simulink model "MyECUModel_OLD"  (R2022a)
settings: Solver=FixedStepAuto  StartTime=0.0  StopTime=1  FixedStep=0.0001  RelTol=1e-3
model workspace (MAT data in the model file):
  rpm = 3000
values from neighbouring files (symbols this model uses):
  AFR = 9.75    [MyECUModel_OLD_Params.m]
  engine_displacement = 0.000599    [MyECUModel_OLD_Params.m]
  fuel_mass_flow_rate = 1    [MyECUModel_OLD_Params.m]
  ignition_1 = 160    [MyECUModel_OLD_Params.m]
  ignition_2 = 250    [MyECUModel_OLD_Params.m]
  ignition_3 = 340    [MyECUModel_OLD_Params.m]
  ignition_4 = 70    [MyECUModel_OLD_Params.m]
  ignition_dwell_time = 0.003    [MyECUModel_OLD_Params.m]
  inj_valve_open_time = 1.134    [MyECUModel_OLD_Params.m]
  injection_duration = 24    [MyECUModel_OLD_Params.m]
  injection_start_1 = 120    [MyECUModel_OLD_Params.m]
  injection_start_2 = 210    [MyECUModel_OLD_Params.m]
  injection_start_3 = 300    [MyECUModel_OLD_Params.m]
  injection_start_4 = 30    [MyECUModel_OLD_Params.m]
  intake_air_temp = 300    [MyECUModel_OLD_Params.m]
  manifold_pressure = 100000    [MyECUModel_OLD_Params.m]
  volumetric_efficiency = 1    [MyECUModel_OLD_Params.m]
libraries: simulink x14
settings Model: Creator=feyzi  LastModifiedBy=feyzi
settings DebuggingCC: UnconnectedInputMsg=warning  UnconnectedOutputMsg=warning  UnconnectedLineMsg=warning
settings HardwareCC: ProdBitPerLong=64  ProdLargestAtomicFloat=None  ProdHWDeviceType=AMD->Athlon 64
settings RTWCC: DLArmComputeVersion=19.05

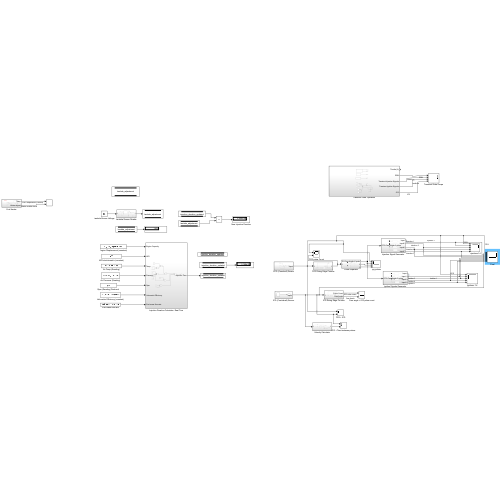
[thumbnail: Simulink's stored preview of the top-level diagram]
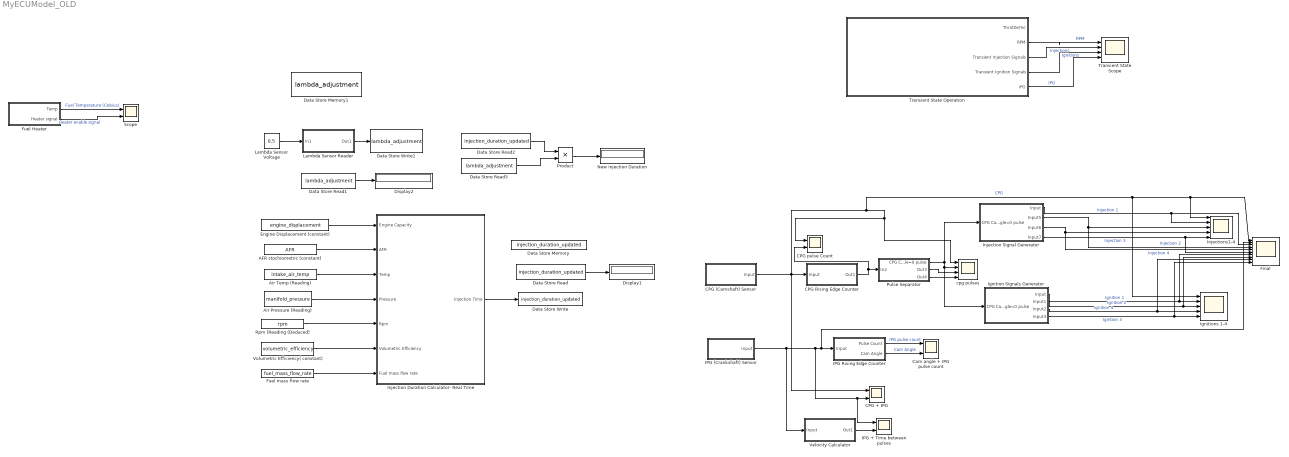
== system MyECUModel_OLD ==
  AFR stochiometric (constant) : Constant  Value=AFR
  Air Pressure (Reading) : Constant  Value=manifold_pressure
  Air Temp (Reading) : Constant  Value=intake_air_temp
  CPG (Camshaft) Sensor : Subsystem
  CPG + IPG : Scope  NumInputPorts=2
  CPG Rising Edge Counter : Subsystem
  CPG pulse Count : Scope  NumInputPorts=2
  Cam angle + IPG pulse count : Scope  NumInputPorts=2
  Data Store Memory : DataStoreMemory  DataStoreName=injection_duration_updated  ReadBeforeWriteMsg=warning  WriteAfterWriteMsg=warning  WriteAfterReadMsg=warning  ShowAdditionalParam=off
  Data Store Memory1 : DataStoreMemory  DataStoreName=lambda_adjustment  ReadBeforeWriteMsg=warning  WriteAfterWriteMsg=warning  WriteAfterReadMsg=warning  ShowAdditionalParam=off
  Data Store Read : DataStoreRead  DataStoreName=injection_duration_updated  IndexOptions=Index vector (dialog)  Indices=1  OutputSizes=1
  Data Store Read1 : DataStoreRead  DataStoreName=lambda_adjustment  IndexOptions=Index vector (dialog)  Indices=1  OutputSizes=1
  Data Store Read2 : DataStoreRead  DataStoreName=injection_duration_updated  IndexOptions=Index vector (dialog)  Indices=1  OutputSizes=1
  Data Store Read3 : DataStoreRead  DataStoreName=lambda_adjustment  IndexOptions=Index vector (dialog)  Indices=1  OutputSizes=1
  Data Store Write : DataStoreWrite  DataStoreName=injection_duration_updated  IndexOptions=Index vector (dialog)  Indices=1  OutputSizes=1
  Data Store Write1 : DataStoreWrite  DataStoreName=lambda_adjustment  IndexOptions=Index vector (dialog)  Indices=1  OutputSizes=1
  Display1 : Display
  Display2 : Display
  Engine Displacement (constant) : Constant  Value=engine_displacement
  Final : Scope  NumInputPorts=10
  Fuel Heater : Subsystem
  Fuel mass flow rate : Constant  Value=fuel_mass_flow_rate
  IPG (Crankshaft) Sensor : Subsystem
  IPG + Time between pulses : Scope  NumInputPorts=2
  IPG Rising Edge Counter : Subsystem
  Ignition Signals Generator : Subsystem
  Ignitions 1-4 : Scope  NumInputPorts=5
  Injection Duration Calculator- Real Time : Subsystem
  Injection Signal Generator : Subsystem
  Injections1-4 : Scope  NumInputPorts=5
  Lambda Sensor Reader : Subsystem
  Lambda Sensor Voltage : Constant  Value=0.5
  New Injection Duration : Display
  Product : Product
  Pulse Separator : Subsystem
  Rpm (Reading (Deduced) : Constant  Value=rpm
  Scope : Scope  NumInputPorts=2
  Transient State Operation : Subsystem
  Transient State Scope : Scope  NumInputPorts=4
  Velocity Calculator : Subsystem
  Volumetric Efficiency( constant) : Constant  Value=volumetric_efficiency
  cpg pulses : Scope  NumInputPorts=4
  wires:
  IPG (Crankshaft) Sensor/1(Input) -> IPG Rising Edge Counter/1(Input), Final/2, CPG + IPG/2, IPG + Time between pulses/1, Velocity Calculator/1(Input)
  CPG (Camshaft) Sensor/1(Input) -> Final/1, Injections1-4/1, Ignitions 1-4/1, cpg pulses/1, CPG pulse Count/1, CPG Rising Edge Counter/1(Input), CPG + IPG/1  "CPG"
  CPG Rising Edge Counter/1(Out1) -> Pulse Separator/1(In2), CPG pulse Count/2
  Pulse Separator/1(CPG Cam Angle=0 pulse) -> Ignition Signals Generator/1(CPG Cam Angle=0 pulse), cpg pulses/2, Injection Signal Generator/1(CPG Cam Angle=0 pulse)
  Pulse Separator/2(Out3) -> cpg pulses/3
  Pulse Separator/3(Out4) -> cpg pulses/4
  Engine Displacement (constant)/1 -> Injection Duration Calculator- Real Time/1(Engine Capacity)
  AFR stochiometric (constant)/1 -> Injection Duration Calculator- Real Time/2(AFR)
  Air Temp (Reading)/1 -> Injection Duration Calculator- Real Time/3(Temp)
  Air Pressure (Reading)/1 -> Injection Duration Calculator- Real Time/4(Pressure)
  Injection Signal Generator/3(Input6) -> Final/5, Injections1-4/4  "Injection 4"
  Injection Signal Generator/2(Input5) -> Injections1-4/3, Final/4  "Injection 2"
  Injection Signal Generator/4(Input7) -> Injections1-4/5, Final/6  "Injection 3"
  Ignition Signals Generator/1(Input) -> Final/7, Ignitions 1-4/2  "Ignition 1"
  Ignition Signals Generator/2(Input1) -> Final/8, Ignitions 1-4/3  "Ignition 2"
  Ignition Signals Generator/3(Input2) -> Final/9, Ignitions 1-4/4  "Ignition 4"
  Ignition Signals Generator/4(Input3) -> Final/10, Ignitions 1-4/5  "Ignition 3"
  Injection Signal Generator/1(Input) -> Injections1-4/2, Final/3  "Injection 1"
  Rpm (Reading (Deduced)/1 -> Injection Duration Calculator- Real Time/5(Rpm)
  Volumetric Efficiency( constant)/1 -> Injection Duration Calculator- Real Time/6(Volumetric Efficiency)
  Fuel mass flow rate/1 -> Injection Duration Calculator- Real Time/7(Fuel mass flow rate)
  Injection Duration Calculator- Real Time/1(Injection Time) -> Data Store Write/1
  IPG Rising Edge Counter/2(Cam Angle) -> Cam angle + IPG pulse count/2  "Cam Angle"
  IPG Rising Edge Counter/1(Pulse Count) -> Cam angle + IPG pulse count/1  "IPG pulse count"
  Data Store Read/1 -> Display1/1
  Lambda Sensor Voltage/1 -> Lambda Sensor Reader/1(In1)
  Lambda Sensor Reader/1(Out1) -> Data Store Write1/1
  Data Store Read1/1 -> Display2/1
  Data Store Read2/1 -> Product/1
  Data Store Read3/1 -> Product/2
  Product/1 -> New Injection Duration/1
  Velocity Calculator/1(Out1) -> IPG + Time between pulses/2
  Transient State Operation/2(RPM) -> Transient State Scope/1  "RPM"
  Transient State Operation/3(Transient Injection Signals) -> Transient State Scope/2  "Injections"
  Transient State Operation/4(Transient Ignition Signals) -> Transient State Scope/3  "Ignitions"
  Transient State Operation/5(ıPG) -> Transient State Scope/4  "IPG"
  Fuel Heater/1(Temp) -> Scope/1  "Fuel Temperature (Celsius)"
  Fuel Heater/2(Heater signal) -> Scope/2  "Heater enable signal"

== system MyECUModel_OLD/CPG (Camshaft) Sensor ==
  Peak 2(Ref) : DiscretePulseGenerator  PulseType=Time based  Period=1  PulseWidth=5  PhaseDelay=0.1
  Peak 3 (TDC- before Power) : DiscretePulseGenerator  PulseType=Time based  Period=1  PulseWidth=5  PhaseDelay=0.5
  Peak1(cycle start - injection TDC) : DiscretePulseGenerator  PulseType=Time based  Period=1  PulseWidth=5
  Sum : Sum  Inputs=|+++  InputSameDT=on
  Unit Delay1 : UnitDelay  SampleTime=-1  HasFrameUpgradeWarning=on
  Input : Outport
  wires:
  Sum/1 -> Unit Delay1/1
  Peak1(cycle start - injection TDC)/1 -> Sum/1
  Peak 2(Ref)/1 -> Sum/2
  Peak 3 (TDC- before Power)/1 -> Sum/3
  Unit Delay1/1 -> Input/1

== system MyECUModel_OLD/CPG Rising Edge Counter ==
  Input : Inport
  Count Resetter : simulink/Logic and Bit Operations/Compare To Constant  relop=>=  const=3.0  OutDataTypeStr=boolean
  Delay : Delay  DelayLength=1
  Detect Rise Positive : simulink/Logic and Bit Operations/Detect Rise Positive  vinit=0  OutDataTypeStr=uint8
  Rising Edge Counter : Subsystem  TreatAsAtomicUnit=on
  Scope : Scope  NumInputPorts=2
  Out1 : Outport
  wires:
  Delay/1 -> Rising Edge Counter/Reset
  Input/1 -> Detect Rise Positive/1, Scope/1  "CPG signal"
  Detect Rise Positive/1 -> Rising Edge Counter/1(In1)  "Rising Edge Detected"
  Count Resetter/1 -> Delay/1
  Rising Edge Counter/1(Out1) -> Out1/1, Scope/2, Count Resetter/1  "CPG Pulse Count"

== system MyECUModel_OLD/Fuel Heater ==
  Ramp : simulink/Sources/Ramp  slope=20  start=0.5  InitialOutput=0
  Ramp1 : simulink/Sources/Ramp  slope=-20  start=2.5  InitialOutput=0
  Step1 : Step  Time=0  Before=30  After=30  SampleTime=0
  Step2 : Step  Time=0.5  SampleTime=0
  Step3 : Step  Time=2.5  After=-1  SampleTime=0
  Sum : Sum  Inputs=|+++
  Sum1 : Sum  Inputs=|++
  Temp : Outport
  Heater signal : Outport  Port=2
  wires:
  ? -> ?
  Step1/1 -> Sum/1
  Ramp/1 -> Sum/2
  Sum/1 -> Temp/1
  Ramp1/1 -> Sum/3
  Step2/1 -> Sum1/2
  Step3/1 -> Sum1/1
  Sum1/1 -> Heater signal/1

== system MyECUModel_OLD/IPG (Crankshaft) Sensor ==
  Pulse Generator : DiscretePulseGenerator  PulseType=Time based  Period=0.042  PulseWidth=5
  Input : Outport
  wires:
  Pulse Generator/1 -> Input/1

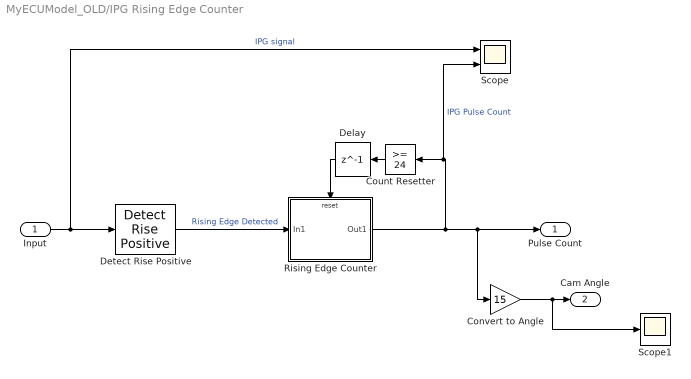
== system MyECUModel_OLD/IPG Rising Edge Counter ==
  Input : Inport
  Convert to Angle : Gain  Gain=15
  Count Resetter : simulink/Logic and Bit Operations/Compare To Constant  relop=>=  const=24  OutDataTypeStr=boolean
  Delay : Delay  DelayLength=1
  Detect Rise Positive : simulink/Logic and Bit Operations/Detect Rise Positive  vinit=0  OutDataTypeStr=uint8
  Rising Edge Counter : Subsystem  TreatAsAtomicUnit=on
  Scope : Scope  NumInputPorts=2
  Scope1 : Scope
  Pulse Count : Outport
  Cam Angle : Outport  Port=2
  wires:
  Delay/1 -> Rising Edge Counter/Reset
  Input/1 -> Detect Rise Positive/1, Scope/1  "IPG signal"
  Detect Rise Positive/1 -> Rising Edge Counter/1(In1)  "Rising Edge Detected"
  Count Resetter/1 -> Delay/1
  Rising Edge Counter/1(Out1) -> Convert to Angle/1, Pulse Count/1, Scope/2, Count Resetter/1  "IPG Pulse Count"
  Convert to Angle/1 -> Scope1/1, Cam Angle/1

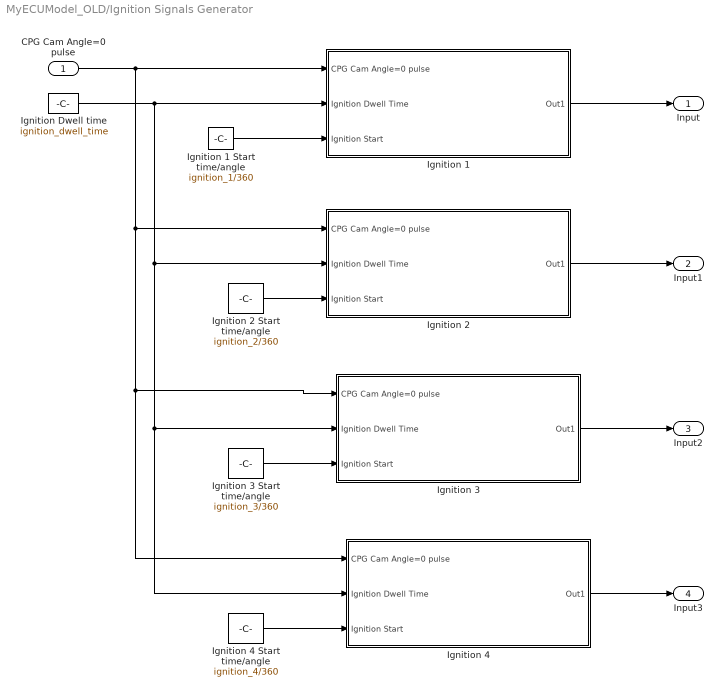
== system MyECUModel_OLD/Ignition Signals Generator ==
  CPG Cam Angle=0 pulse : Inport
  Ignition 1 : Subsystem
  Ignition 1 Start time/angle : Constant  Value=ignition_1/360
  Ignition 2 : Subsystem
  Ignition 2 Start time/angle : Constant  Value=ignition_2/360
  Ignition 3 : Subsystem
  Ignition 3 Start time/angle : Constant  Value=ignition_3/360
  Ignition 4 : Subsystem
  Ignition 4 Start time/angle : Constant  Value=ignition_4/360
  Ignition Dwell time : Constant  Value=ignition_dwell_time
  Input : Outport
  Input1 : Outport  Port=2
  Input2 : Outport  Port=3
  Input3 : Outport  Port=4
  wires:
  CPG Cam Angle=0 pulse/1 -> Ignition 2/1(CPG Cam Angle=0 pulse), Ignition 4/1(CPG Cam Angle=0 pulse), Ignition 3/1(CPG Cam Angle=0 pulse), Ignition 1/1(CPG Cam Angle=0 pulse)
  Ignition Dwell time/1 -> Ignition 2/2(Ignition Dwell Time), Ignition 4/2(Ignition Dwell Time), Ignition 3/2(Ignition Dwell Time), Ignition 1/2(Ignition Dwell Time)
  Ignition 1 Start time/angle/1 -> Ignition 1/3(Ignition Start)
  Ignition 1/1(Out1) -> Input/1
  Ignition 2/1(Out1) -> Input1/1
  Ignition 3/1(Out1) -> Input2/1
  Ignition 4/1(Out1) -> Input3/1
  Ignition 2 Start time/angle/1 -> Ignition 2/3(Ignition Start)
  Ignition 3 Start time/angle/1 -> Ignition 3/3(Ignition Start)
  Ignition 4 Start time/angle/1 -> Ignition 4/3(Ignition Start)

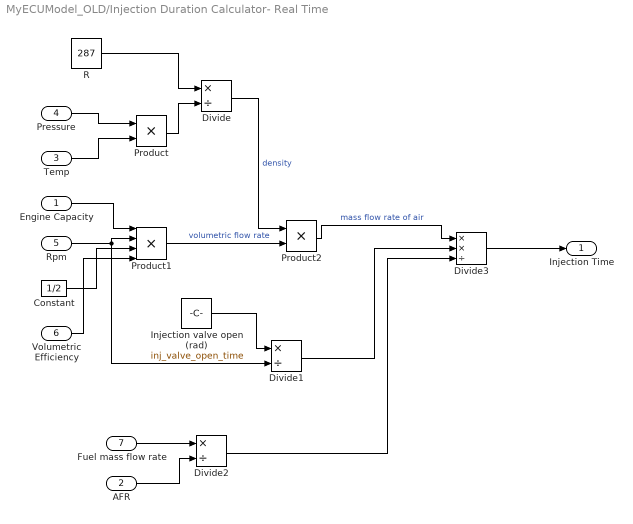
== system MyECUModel_OLD/Injection Duration Calculator- Real Time ==
  Engine Capacity : Inport
  AFR : Inport  Port=2
  Temp : Inport  Port=3
  Pressure : Inport  Port=4
  Rpm : Inport  Port=5
  Volumetric Efficiency : Inport  Port=6
  Fuel mass flow rate : Inport  Port=7
  Constant : Constant  Value=1/2
  Divide : Product  Inputs=*/
  Divide1 : Product  Inputs=*/
  Divide2 : Product  Inputs=*/
  Divide3 : Product  Inputs=**/
  Injection valve open (rad) : Constant  Value=inj_valve_open_time
  Product : Product
  Product1 : Product  Inputs=4
  Product2 : Product
  R : Constant  Value=287
  Injection Time : Outport
  wires:
  Pressure/1 -> Product/1
  Temp/1 -> Product/2
  R/1 -> Divide/1
  Product/1 -> Divide/2
  Divide/1 -> Product2/1  "density"
  Engine Capacity/1 -> Product1/1
  Rpm/1 -> Divide1/2, Product1/2
  Constant/1 -> Product1/3
  Product1/1 -> Product2/2  "volumetric flow rate"
  Product2/1 -> Divide3/1  "mass flow rate of air"
  Injection valve open (rad)/1 -> Divide1/1
  Fuel mass flow rate/1 -> Divide2/1
  AFR/1 -> Divide2/2
  Volumetric Efficiency/1 -> Product1/4
  Divide2/1 -> Divide3/3
  Divide1/1 -> Divide3/2
  Divide3/1 -> Injection Time/1

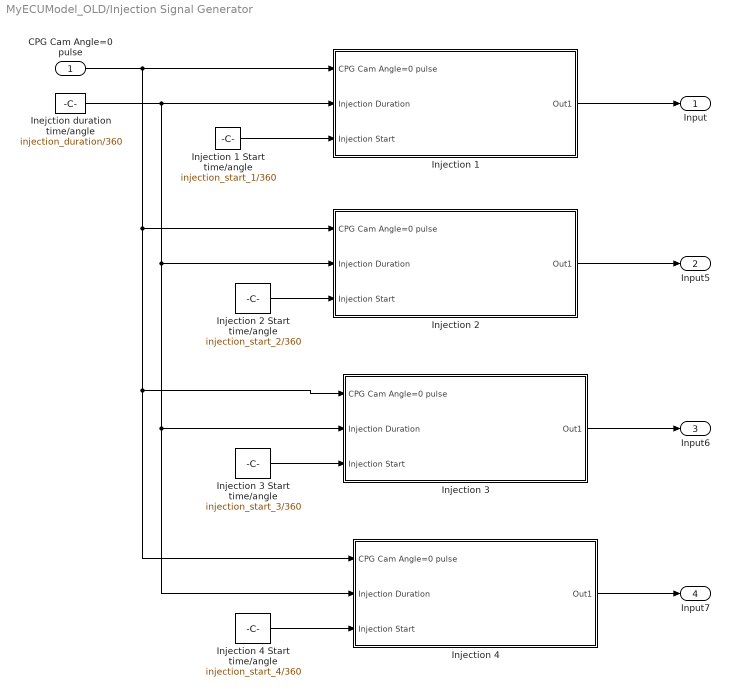
== system MyECUModel_OLD/Injection Signal Generator ==
  CPG Cam Angle=0 pulse : Inport
  Inejction duration time/angle : Constant  Value=injection_duration/360
  Injection 1 : Subsystem
  Injection 1 Start time/angle : Constant  Value=injection_start_1/360
  Injection 2 : Subsystem
  Injection 2 Start time/angle : Constant  Value=injection_start_2/360
  Injection 3 : Subsystem
  Injection 3 Start time/angle : Constant  Value=injection_start_3/360
  Injection 4 : Subsystem
  Injection 4 Start time/angle : Constant  Value=injection_start_4/360
  Input : Outport
  Input5 : Outport  Port=2
  Input6 : Outport  Port=3
  Input7 : Outport  Port=4
  wires:
  CPG Cam Angle=0 pulse/1 -> Injection 3/1(CPG Cam Angle=0 pulse), Injection 4/1(CPG Cam Angle=0 pulse), Injection 2/1(CPG Cam Angle=0 pulse), Injection 1/1(CPG Cam Angle=0 pulse)
  Inejction duration time/angle/1 -> Injection 4/2(Injection Duration), Injection 3/2(Injection Duration), Injection 2/2(Injection Duration), Injection 1/2(Injection Duration)
  Injection 1 Start time/angle/1 -> Injection 1/3(Injection Start)
  Injection 1/1(Out1) -> Input/1
  Injection 2/1(Out1) -> Input5/1
  Injection 3/1(Out1) -> Input6/1
  Injection 4/1(Out1) -> Input7/1
  Injection 2 Start time/angle/1 -> Injection 2/3(Injection Start)
  Injection 3 Start time/angle/1 -> Injection 3/3(Injection Start)
  Injection 4 Start time/angle/1 -> Injection 4/3(Injection Start)

== system MyECUModel_OLD/Lambda Sensor Reader ==
  In1 : Inport
  AFR-Actual : Display
  AFRs : Constant  Value=[19:-0.5:9]
  Constant : Constant  Value=AFR
  Divide : Product  Inputs=/*
  Lookup Table Dynamic : simulink/Lookup Tables/Lookup Table Dynamic  LookUpMeth=Interpolation-Use End Values  OutDataType=fixdt('double')  OutScaling=[]  OutputDataTypeScalingMode=Specify via dialog  OutDataTypeStr=double  DoSatur=off
  Voltages : Constant  Value=[0:0.05:1]
  Out1 : Outport
  wires:
  In1/1 -> Lookup Table Dynamic/1
  Voltages/1 -> Lookup Table Dynamic/2
  AFRs/1 -> Lookup Table Dynamic/3
  Lookup Table Dynamic/1 -> AFR-Actual/1, Divide/2
  Divide/1 -> Out1/1
  Constant/1 -> Divide/1

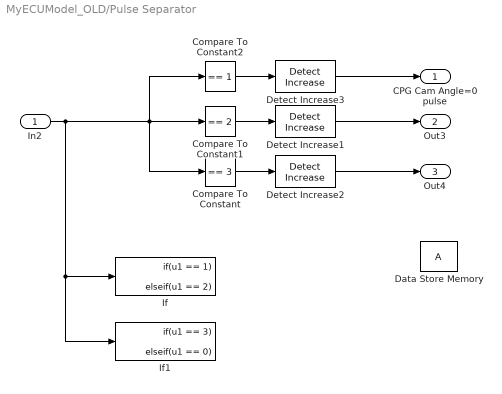
== system MyECUModel_OLD/Pulse Separator ==
  In2 : Inport
  Compare To Constant : simulink/Logic and Bit Operations/Compare To Constant  relop===  const=3  OutDataTypeStr=uint8
  Compare To Constant1 : simulink/Logic and Bit Operations/Compare To Constant  relop===  const=2  OutDataTypeStr=uint8
  Compare To Constant2 : simulink/Logic and Bit Operations/Compare To Constant  relop===  const=1  OutDataTypeStr=uint8
  Data Store Memory : DataStoreMemory  ReadBeforeWriteMsg=warning  WriteAfterWriteMsg=warning  WriteAfterReadMsg=warning  ShareAcrossModelInstances=on  ShowAdditionalParam=off  OutMin=0  OutMax=12
  Detect Increase1 : simulink/Logic and Bit Operations/Detect Increase  vinit=0.0  OutDataTypeStr=uint8
  Detect Increase2 : simulink/Logic and Bit Operations/Detect Increase  vinit=0.0  OutDataTypeStr=uint8
  Detect Increase3 : simulink/Logic and Bit Operations/Detect Increase  vinit=0.0  OutDataTypeStr=uint8
  If : If  IfExpression=u1 == 1  ElseIfExpressions=u1 == 2  ShowElse=off
  If1 : If  IfExpression=u1 == 3  ElseIfExpressions=u1 == 0  ShowElse=off
  CPG Cam Angle=0 pulse : Outport  OutDataTypeStr=uint8
  Out3 : Outport  Port=2
  Out4 : Outport  Port=3
  wires:
  Detect Increase2/1 -> Out4/1
  In2/1 -> If1/1, If/1, Compare To Constant2/1, Compare To Constant/1, Compare To Constant1/1
  Compare To Constant1/1 -> Detect Increase1/1
  Detect Increase1/1 -> Out3/1
  Compare To Constant/1 -> Detect Increase2/1
  Compare To Constant2/1 -> Detect Increase3/1
  Detect Increase3/1 -> CPG Cam Angle=0 pulse/1

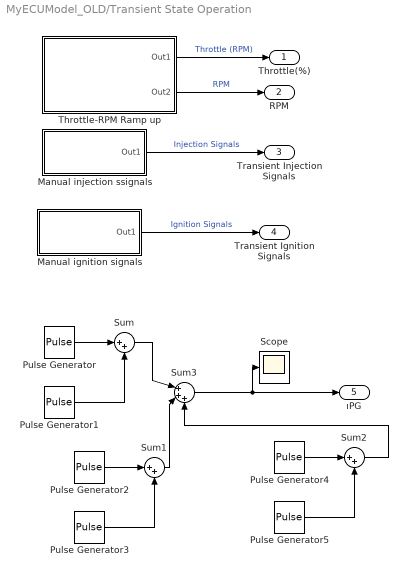
== system MyECUModel_OLD/Transient State Operation ==
  Manual ignition signals : Subsystem
  Manual injection ssignals : Subsystem
  Pulse Generator : DiscretePulseGenerator  PulseType=Time based  Period=0.1  PulseWidth=5
  Pulse Generator1 : DiscretePulseGenerator  PulseType=Time based  Amplitude=-1  Period=0.1  PulseWidth=5  PhaseDelay=1
  Pulse Generator2 : DiscretePulseGenerator  PulseType=Time based  Period=0.08  PulseWidth=5  PhaseDelay=1
  Pulse Generator3 : DiscretePulseGenerator  PulseType=Time based  Amplitude=-1  Period=0.08  PulseWidth=5  PhaseDelay=1.96
  Pulse Generator4 : DiscretePulseGenerator  PulseType=Time based  Period=0.06  PulseWidth=5  PhaseDelay=1.96
  Pulse Generator5 : DiscretePulseGenerator  PulseType=Time based  Amplitude=-1  Period=0.06  PulseWidth=5  PhaseDelay=3
  Scope : Scope
  Sum : Sum  Inputs=|++
  Sum1 : Sum  Inputs=|++
  Sum2 : Sum  Inputs=|++
  Sum3 : Sum  Inputs=|+++
  Throttle-RPM Ramp up : Subsystem
  Throttle(%) : Outport
  RPM : Outport  Port=2
  Transient Injection Signals : Outport  Port=3
  Transient Ignition Signals : Outport  Port=4
  ıPG : Outport  Port=5
  wires:
  Throttle-RPM Ramp up/2(Out2) -> RPM/1  "RPM"
  Throttle-RPM Ramp up/1(Out1) -> Throttle(%)/1  "Throttle (RPM)"
  Manual injection ssignals/1(Out1) -> Transient Injection Signals/1  "Injection Signals"
  Manual ignition signals/1(Out1) -> Transient Ignition Signals/1  "Ignition Signals"
  Pulse Generator/1 -> Sum/1
  Pulse Generator1/1 -> Sum/2
  Sum/1 -> Sum3/1
  Pulse Generator2/1 -> Sum1/1
  Pulse Generator3/1 -> Sum1/2
  Pulse Generator4/1 -> Sum2/1
  Pulse Generator5/1 -> Sum2/2
  Sum2/1 -> Sum3/3
  Sum1/1 -> Sum3/2
  Sum3/1 -> Scope/1, ıPG/1

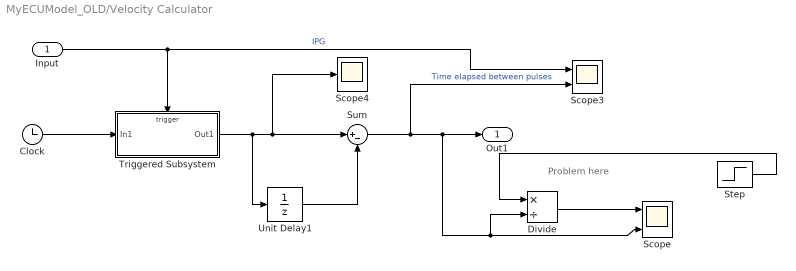
== system MyECUModel_OLD/Velocity Calculator ==
  note: Problem here
  Input : Inport
  Clock : Clock
      settings: Decimation=100
  Divide : Product  Inputs=*/
  Scope : Scope  NumInputPorts=2
  Scope3 : Scope  NumInputPorts=2
  Scope4 : Scope
  Step : Step  Time=0  After=30/12  SampleTime=0
  Sum : Sum  Inputs=|+-
  Triggered Subsystem : Subsystem  TreatAsAtomicUnit=on
  Unit Delay1 : UnitDelay  SampleTime=-1
  Out1 : Outport
  wires:
  Sum/1 -> Scope3/2, Divide/2, Scope/2, Out1/1  "Time elapsed between pulses"
  Input/1 -> Scope3/1, Triggered Subsystem/Trigger  "IPG"
  Unit Delay1/1 -> Sum/2
  Clock/1 -> Triggered Subsystem/1(In1)
  Triggered Subsystem/1(Out1) -> Sum/1, Scope4/1, Unit Delay1/1
  Step/1 -> Divide/1
  Divide/1 -> Scope/1

== system MyECUModel_OLD/CPG Rising Edge Counter/Rising Edge Counter ==
  In1 : Inport
  Reset : ResetPort  DisableCoverage=on
  Memory : Memory
  Sum1 : Sum  Inputs=|++
  Out1 : Outport
  wires:
  Memory/1 -> Sum1/2
  Sum1/1 -> Out1/1, Memory/1
  In1/1 -> Sum1/1

== system MyECUModel_OLD/IPG Rising Edge Counter/Rising Edge Counter ==
  In1 : Inport
  Reset : ResetPort  DisableCoverage=on
  Memory : Memory
  Sum1 : Sum  Inputs=|++
  Out1 : Outport
  wires:
  Memory/1 -> Sum1/2
  Sum1/1 -> Out1/1, Memory/1
  In1/1 -> Sum1/1

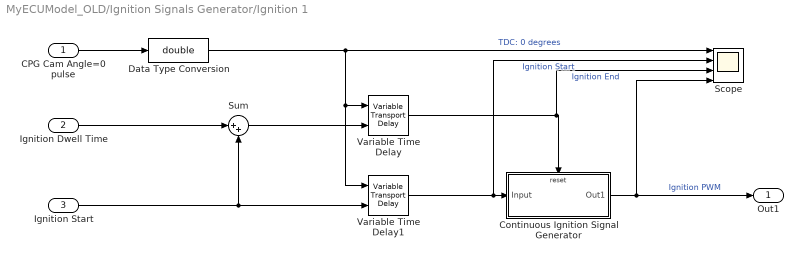
== system MyECUModel_OLD/Ignition Signals Generator/Ignition 1 ==
  CPG Cam Angle=0 pulse : Inport
  Ignition Dwell Time : Inport  Port=2
  Ignition Start : Inport  Port=3
  Continuous Ignition Signal Generator : Subsystem  TreatAsAtomicUnit=on
  Data Type Conversion : DataTypeConversion  OutDataTypeStr=double  SaturateOnIntegerOverflow=off  RndMeth=Floor
  Scope : Scope  NumInputPorts=4
  Sum : Sum  Inputs=|++
  Variable Time Delay : VariableTransportDelay  MaximumDelay=10  MaximumPoints=20480  ZeroDelay=on
  Variable Time Delay1 : VariableTransportDelay  MaximumDelay=10  MaximumPoints=20480  ZeroDelay=on
  Out1 : Outport
  wires:
  Continuous Ignition Signal Generator/1(Out1) -> Scope/4, Out1/1  "Ignition PWM"
  Variable Time Delay/1 -> Scope/3, Continuous Ignition Signal Generator/Reset  "Ignition End"
  Ignition Start/1 -> Sum/2, Variable Time Delay1/2
  CPG Cam Angle=0 pulse/1 -> Data Type Conversion/1
  Variable Time Delay1/1 -> Scope/2, Continuous Ignition Signal Generator/1(Input)  "Ignition Start"
  Data Type Conversion/1 -> Scope/1, Variable Time Delay1/1, Variable Time Delay/1  "TDC: 0 degrees"
  Ignition Dwell Time/1 -> Sum/1
  Sum/1 -> Variable Time Delay/2

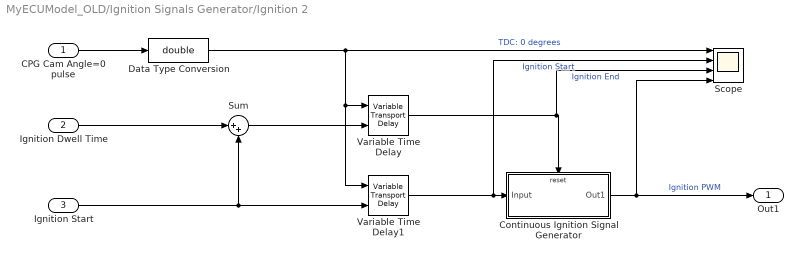
== system MyECUModel_OLD/Ignition Signals Generator/Ignition 2 ==
  CPG Cam Angle=0 pulse : Inport
  Ignition Dwell Time : Inport  Port=2
  Ignition Start : Inport  Port=3
  Continuous Ignition Signal Generator : Subsystem  TreatAsAtomicUnit=on
  Data Type Conversion : DataTypeConversion  OutDataTypeStr=double  SaturateOnIntegerOverflow=off  RndMeth=Floor
  Scope : Scope  NumInputPorts=4
  Sum : Sum  Inputs=|++
  Variable Time Delay : VariableTransportDelay  MaximumDelay=10  MaximumPoints=20480  ZeroDelay=on
  Variable Time Delay1 : VariableTransportDelay  MaximumDelay=10  MaximumPoints=20480  ZeroDelay=on
  Out1 : Outport
  wires:
  Continuous Ignition Signal Generator/1(Out1) -> Scope/4, Out1/1  "Ignition PWM"
  Variable Time Delay/1 -> Scope/3, Continuous Ignition Signal Generator/Reset  "Ignition End"
  Ignition Start/1 -> Sum/2, Variable Time Delay1/2
  CPG Cam Angle=0 pulse/1 -> Data Type Conversion/1
  Variable Time Delay1/1 -> Scope/2, Continuous Ignition Signal Generator/1(Input)  "Ignition Start"
  Data Type Conversion/1 -> Scope/1, Variable Time Delay1/1, Variable Time Delay/1  "TDC: 0 degrees"
  Ignition Dwell Time/1 -> Sum/1
  Sum/1 -> Variable Time Delay/2

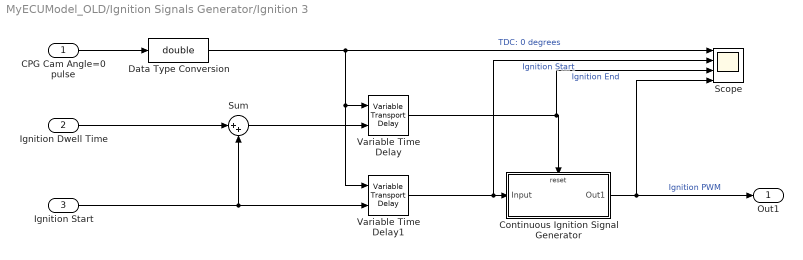
== system MyECUModel_OLD/Ignition Signals Generator/Ignition 3 ==
  CPG Cam Angle=0 pulse : Inport
  Ignition Dwell Time : Inport  Port=2
  Ignition Start : Inport  Port=3
  Continuous Ignition Signal Generator : Subsystem  TreatAsAtomicUnit=on
  Data Type Conversion : DataTypeConversion  OutDataTypeStr=double  SaturateOnIntegerOverflow=off  RndMeth=Floor
  Scope : Scope  NumInputPorts=4
  Sum : Sum  Inputs=|++
  Variable Time Delay : VariableTransportDelay  MaximumDelay=10  MaximumPoints=20480  ZeroDelay=on
  Variable Time Delay1 : VariableTransportDelay  MaximumDelay=10  MaximumPoints=20480  ZeroDelay=on
  Out1 : Outport
  wires:
  Continuous Ignition Signal Generator/1(Out1) -> Scope/4, Out1/1  "Ignition PWM"
  Variable Time Delay/1 -> Scope/3, Continuous Ignition Signal Generator/Reset  "Ignition End"
  Ignition Start/1 -> Sum/2, Variable Time Delay1/2
  CPG Cam Angle=0 pulse/1 -> Data Type Conversion/1
  Variable Time Delay1/1 -> Scope/2, Continuous Ignition Signal Generator/1(Input)  "Ignition Start"
  Data Type Conversion/1 -> Scope/1, Variable Time Delay1/1, Variable Time Delay/1  "TDC: 0 degrees"
  Ignition Dwell Time/1 -> Sum/1
  Sum/1 -> Variable Time Delay/2

== system MyECUModel_OLD/Ignition Signals Generator/Ignition 4 ==
  CPG Cam Angle=0 pulse : Inport
  Ignition Dwell Time : Inport  Port=2
  Ignition Start : Inport  Port=3
  Continuous Ignition Signal Generator : Subsystem  TreatAsAtomicUnit=on
  Data Type Conversion : DataTypeConversion  OutDataTypeStr=double  SaturateOnIntegerOverflow=off  RndMeth=Floor
  Scope : Scope  NumInputPorts=4
  Sum : Sum  Inputs=|++
  Variable Time Delay : VariableTransportDelay  MaximumDelay=10  MaximumPoints=20480  ZeroDelay=on
  Variable Time Delay1 : VariableTransportDelay  MaximumDelay=10  MaximumPoints=20480  ZeroDelay=on
  Out1 : Outport
  wires:
  Continuous Ignition Signal Generator/1(Out1) -> Scope/4, Out1/1  "Ignition PWM"
  Variable Time Delay/1 -> Scope/3, Continuous Ignition Signal Generator/Reset  "Ignition End"
  Ignition Start/1 -> Variable Time Delay1/2, Sum/2
  CPG Cam Angle=0 pulse/1 -> Data Type Conversion/1
  Variable Time Delay1/1 -> Scope/2, Continuous Ignition Signal Generator/1(Input)  "Ignition Start"
  Data Type Conversion/1 -> Scope/1, Variable Time Delay1/1, Variable Time Delay/1  "TDC: 0 degrees"
  Ignition Dwell Time/1 -> Sum/1
  Sum/1 -> Variable Time Delay/2

== system MyECUModel_OLD/Injection Signal Generator/Injection 1 ==
  CPG Cam Angle=0 pulse : Inport
  Injection Duration : Inport  Port=2
  Injection Start : Inport  Port=3
  Continuous Injection Signal Generator : Subsystem  TreatAsAtomicUnit=on
  Data Type Conversion : DataTypeConversion  OutDataTypeStr=double  SaturateOnIntegerOverflow=off  RndMeth=Floor
  Scope : Scope  NumInputPorts=4
  Sum : Sum  Inputs=|++
  Variable Time Delay : VariableTransportDelay  MaximumDelay=10  MaximumPoints=20480  ZeroDelay=on
  Variable Time Delay1 : VariableTransportDelay  MaximumDelay=10  MaximumPoints=30720  ZeroDelay=on
  Out1 : Outport
  wires:
  Continuous Injection Signal Generator/1(Out1) -> Scope/4, Out1/1  "Injection 1 pwm"
  Variable Time Delay/1 -> Scope/3, Continuous Injection Signal Generator/Reset  "Injection 1 end"
  Injection Start/1 -> Sum/2, Variable Time Delay1/2
  CPG Cam Angle=0 pulse/1 -> Data Type Conversion/1
  Variable Time Delay1/1 -> Scope/2, Continuous Injection Signal Generator/1(Input)  "Injection 1 start"
  Data Type Conversion/1 -> Scope/1, Variable Time Delay1/1, Variable Time Delay/1  "TDC: 0 degrees"
  Injection Duration/1 -> Sum/1
  Sum/1 -> Variable Time Delay/2

== system MyECUModel_OLD/Injection Signal Generator/Injection 2 ==
  CPG Cam Angle=0 pulse : Inport
  Injection Duration : Inport  Port=2
  Injection Start : Inport  Port=3
  Continuous Injection Signal Generator : Subsystem  TreatAsAtomicUnit=on
  Data Type Conversion : DataTypeConversion  OutDataTypeStr=double  SaturateOnIntegerOverflow=off  RndMeth=Floor
  Scope : Scope  NumInputPorts=4
  Sum : Sum  Inputs=|++
  Variable Time Delay : VariableTransportDelay  MaximumDelay=10  MaximumPoints=20480  ZeroDelay=on
  Variable Time Delay1 : VariableTransportDelay  MaximumDelay=10  MaximumPoints=30720  ZeroDelay=on
  Out1 : Outport
  wires:
  Continuous Injection Signal Generator/1(Out1) -> Scope/4, Out1/1  "Injection 2 pwm"
  Variable Time Delay/1 -> Scope/3, Continuous Injection Signal Generator/Reset  "Injection 2 end"
  Injection Start/1 -> Sum/2, Variable Time Delay1/2
  CPG Cam Angle=0 pulse/1 -> Data Type Conversion/1
  Variable Time Delay1/1 -> Scope/2, Continuous Injection Signal Generator/1(Input)  "Injection 2 start"
  Data Type Conversion/1 -> Scope/1, Variable Time Delay1/1, Variable Time Delay/1  "TDC: 0 degrees"
  Injection Duration/1 -> Sum/1
  Sum/1 -> Variable Time Delay/2

== system MyECUModel_OLD/Injection Signal Generator/Injection 3 ==
  CPG Cam Angle=0 pulse : Inport
  Injection Duration : Inport  Port=2
  Injection Start : Inport  Port=3
  Continuous Injection Signal Generator : Subsystem  TreatAsAtomicUnit=on
  Data Type Conversion : DataTypeConversion  OutDataTypeStr=double  SaturateOnIntegerOverflow=off  RndMeth=Floor
  Scope : Scope  NumInputPorts=4
  Sum : Sum  Inputs=|++
  Variable Time Delay : VariableTransportDelay  MaximumDelay=10  MaximumPoints=20480  ZeroDelay=on
  Variable Time Delay1 : VariableTransportDelay  MaximumDelay=10  MaximumPoints=20480  ZeroDelay=on
  Out1 : Outport
  wires:
  Continuous Injection Signal Generator/1(Out1) -> Scope/4, Out1/1  "Injection 3 pwm"
  Variable Time Delay/1 -> Scope/3, Continuous Injection Signal Generator/Reset  "Injection 3 end"
  Injection Start/1 -> Sum/2, Variable Time Delay1/2
  CPG Cam Angle=0 pulse/1 -> Data Type Conversion/1
  Variable Time Delay1/1 -> Scope/2, Continuous Injection Signal Generator/1(Input)  "Injection 3 start"
  Data Type Conversion/1 -> Scope/1, Variable Time Delay1/1, Variable Time Delay/1  "TDC: 0 degrees"
  Injection Duration/1 -> Sum/1
  Sum/1 -> Variable Time Delay/2

== system MyECUModel_OLD/Injection Signal Generator/Injection 4 ==
  CPG Cam Angle=0 pulse : Inport
  Injection Duration : Inport  Port=2
  Injection Start : Inport  Port=3
  Continuous Injection Signal Generator : Subsystem  TreatAsAtomicUnit=on
  Data Type Conversion : DataTypeConversion  OutDataTypeStr=double  SaturateOnIntegerOverflow=off  RndMeth=Floor
  Scope : Scope  NumInputPorts=4
  Sum : Sum  Inputs=|++
  Variable Time Delay : VariableTransportDelay  MaximumDelay=10  MaximumPoints=20480  ZeroDelay=on
  Variable Time Delay1 : VariableTransportDelay  MaximumDelay=10  MaximumPoints=20480  ZeroDelay=on
  Out1 : Outport
  wires:
  Continuous Injection Signal Generator/1(Out1) -> Scope/4, Out1/1  "Injection 4 pwm"
  Variable Time Delay/1 -> Scope/3, Continuous Injection Signal Generator/Reset  "Injection 4 end"
  Injection Start/1 -> Sum/2, Variable Time Delay1/2
  CPG Cam Angle=0 pulse/1 -> Data Type Conversion/1
  Variable Time Delay1/1 -> Scope/2, Continuous Injection Signal Generator/1(Input)  "Injection 4 start"
  Data Type Conversion/1 -> Scope/1, Variable Time Delay1/1, Variable Time Delay/1  "TDC: 0 degrees"
  Injection Duration/1 -> Sum/1
  Sum/1 -> Variable Time Delay/2

== system MyECUModel_OLD/Transient State Operation/Manual ignition signals ==
  Add : Sum  Inputs=++++++++
  Pulse Generator : DiscretePulseGenerator  PulseType=Time based  Period=5  PhaseDelay=0.01
  Pulse Generator1 : DiscretePulseGenerator  PulseType=Time based  Period=5  PhaseDelay=0.7
  Pulse Generator2 : DiscretePulseGenerator  PulseType=Time based  Period=5  PhaseDelay=1.3
  Pulse Generator3 : DiscretePulseGenerator  PulseType=Time based  Period=5  PhaseDelay=1.8
  Pulse Generator4 : DiscretePulseGenerator  PulseType=Time based  Period=5  PhaseDelay=2.7
  Pulse Generator5 : DiscretePulseGenerator  PulseType=Time based  Period=5  PhaseDelay=2.2
  Pulse Generator6 : DiscretePulseGenerator  PulseType=Time based  Period=5  PhaseDelay=2.85
  Pulse Generator7 : DiscretePulseGenerator  PulseType=Time based  Period=5  PhaseDelay=2.5
  Out1 : Outport
  wires:
  Pulse Generator/1 -> Add/1
  Pulse Generator1/1 -> Add/2
  Pulse Generator2/1 -> Add/3
  Pulse Generator3/1 -> Add/4
  Pulse Generator5/1 -> Add/5
  Pulse Generator7/1 -> Add/6
  Pulse Generator4/1 -> Add/7
  Pulse Generator6/1 -> Add/8
  Add/1 -> Out1/1

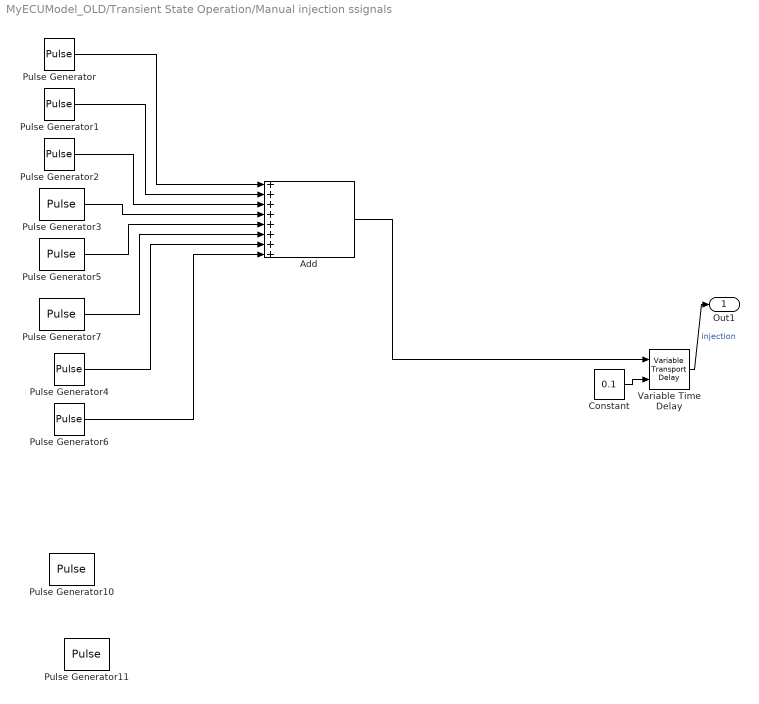
== system MyECUModel_OLD/Transient State Operation/Manual injection ssignals ==
  Add : Sum  Inputs=++++++++
  Constant : Constant  Value=0.1
  Pulse Generator : DiscretePulseGenerator  PulseType=Time based  Period=10
  Pulse Generator1 : DiscretePulseGenerator  PulseType=Time based  Period=10  PhaseDelay=0.7
  Pulse Generator10 : DiscretePulseGenerator  PulseType=Time based  Period=10  PhaseDelay=1.55
  Pulse Generator11 : DiscretePulseGenerator  PulseType=Time based  Period=10  PhaseDelay=1.7
  Pulse Generator2 : DiscretePulseGenerator  PulseType=Time based  Period=10  PhaseDelay=1.3
  Pulse Generator3 : DiscretePulseGenerator  PulseType=Time based  Period=10  PhaseDelay=1.8
  Pulse Generator4 : DiscretePulseGenerator  PulseType=Time based  Period=10  PhaseDelay=2.7
  Pulse Generator5 : DiscretePulseGenerator  PulseType=Time based  Period=10  PhaseDelay=2.2
  Pulse Generator6 : DiscretePulseGenerator  PulseType=Time based  Period=10  PhaseDelay=2.85
  Pulse Generator7 : DiscretePulseGenerator  PulseType=Time based  Period=10  PhaseDelay=2.5
  Variable Time Delay : VariableTransportDelay  MaximumDelay=10
  Out1 : Outport
  wires:
  Pulse Generator/1 -> Add/1
  Pulse Generator1/1 -> Add/2
  Pulse Generator2/1 -> Add/3
  Pulse Generator3/1 -> Add/4
  Pulse Generator5/1 -> Add/5
  Pulse Generator7/1 -> Add/6
  Pulse Generator4/1 -> Add/7
  Pulse Generator6/1 -> Add/8
  Add/1 -> Variable Time Delay/1
  Constant/1 -> Variable Time Delay/2
  Variable Time Delay/1 -> Out1/1  "injection"

== system MyECUModel_OLD/Transient State Operation/Throttle-RPM Ramp up ==
  Gain : Gain  Gain=11000
  Saturation : Saturate  UpperLimit=3000  LowerLimit=0
  Saturation1 : Saturate  UpperLimit=3000/11000  LowerLimit=0
  Scope : Scope  NumInputPorts=2
  Throttle Ramp : simulink/Sources/Ramp  slope=1/10  start=0  InitialOutput=0
  Out1 : Outport
  Out2 : Outport  Port=2
  wires:
  Throttle Ramp/1 -> Saturation1/1, Gain/1
  Gain/1 -> Saturation/1
  Saturation/1 -> Out2/1, Scope/2  "RPM"
  Saturation1/1 -> Out1/1, Scope/1  "Throttle open (%)"

== system MyECUModel_OLD/Velocity Calculator/Triggered Subsystem ==
  In1 : Inport
  Trigger : TriggerPort  VariantControl=(inherit)
  Out1 : Outport
  wires:
  In1/1 -> Out1/1

== system MyECUModel_OLD/Ignition Signals Generator/Ignition 1/Continuous Ignition Signal Generator ==
  Input : Inport
  Reset : ResetPort  DisableCoverage=on
  Memory1 : Memory
  Sum1 : Sum  Inputs=|++
  Out1 : Outport
  wires:
  Sum1/1 -> Out1/1, Memory1/1
  Input/1 -> Sum1/1
  Memory1/1 -> Sum1/2

== system MyECUModel_OLD/Ignition Signals Generator/Ignition 2/Continuous Ignition Signal Generator ==
  Input : Inport
  Reset : ResetPort  DisableCoverage=on
  Memory1 : Memory
  Sum1 : Sum  Inputs=|++
  Out1 : Outport
  wires:
  Sum1/1 -> Out1/1, Memory1/1
  Input/1 -> Sum1/1
  Memory1/1 -> Sum1/2

== system MyECUModel_OLD/Ignition Signals Generator/Ignition 3/Continuous Ignition Signal Generator ==
  Input : Inport
  Reset : ResetPort  DisableCoverage=on
  Memory1 : Memory
  Sum1 : Sum  Inputs=|++
  Out1 : Outport
  wires:
  Sum1/1 -> Out1/1, Memory1/1
  Input/1 -> Sum1/1
  Memory1/1 -> Sum1/2

== system MyECUModel_OLD/Ignition Signals Generator/Ignition 4/Continuous Ignition Signal Generator ==
  Input : Inport
  Reset : ResetPort  DisableCoverage=on
  Memory1 : Memory
  Sum1 : Sum  Inputs=|++
  Out1 : Outport
  wires:
  Sum1/1 -> Out1/1, Memory1/1
  Input/1 -> Sum1/1
  Memory1/1 -> Sum1/2

== system MyECUModel_OLD/Injection Signal Generator/Injection 1/Continuous Injection Signal Generator ==
  Input : Inport
  Reset : ResetPort  DisableCoverage=on
  Memory1 : Memory
  Sum1 : Sum  Inputs=|++
  Out1 : Outport
  wires:
  Sum1/1 -> Out1/1, Memory1/1
  Input/1 -> Sum1/1
  Memory1/1 -> Sum1/2

== system MyECUModel_OLD/Injection Signal Generator/Injection 2/Continuous Injection Signal Generator ==
  Input : Inport
  Reset : ResetPort  DisableCoverage=on
  Memory1 : Memory
  Sum1 : Sum  Inputs=|++
  Out1 : Outport
  wires:
  Sum1/1 -> Out1/1, Memory1/1
  Input/1 -> Sum1/1
  Memory1/1 -> Sum1/2

== system MyECUModel_OLD/Injection Signal Generator/Injection 3/Continuous Injection Signal Generator ==
  Input : Inport
  Reset : ResetPort  DisableCoverage=on
  Memory1 : Memory
  Sum1 : Sum  Inputs=|++
  Out1 : Outport
  wires:
  Sum1/1 -> Out1/1, Memory1/1
  Input/1 -> Sum1/1
  Memory1/1 -> Sum1/2

== system MyECUModel_OLD/Injection Signal Generator/Injection 4/Continuous Injection Signal Generator ==
  Input : Inport
  Reset : ResetPort  DisableCoverage=on
  Memory1 : Memory
  Sum1 : Sum  Inputs=|++
  Out1 : Outport
  wires:
  Sum1/1 -> Out1/1, Memory1/1
  Input/1 -> Sum1/1
  Memory1/1 -> Sum1/2
